simulink model "Spacecraft_ADCS (1)"  (R2017a)
settings: Solver=ode45  StartTime=0.0  StopTime=1000  RelTol=1e-7
values from neighbouring files (symbols this model uses):
  adr = ADRblockGen(w,m,3)    [Example__simulaltion (1).m]    (also in Example__simulaltion.m; WBC_setup (1).m)
  adr2 = ADRblockGen(w2,m,3)    [WBC_setup (1).m]
  aerodrag_A_d = 0.2*0.1*sqrt(2)    [Satellite_Setup_Sun_Pointing (1).m]    (also in Satellite_Setup_Sun_Pointing.m; Satellite_setup_ZenithPointing (1).m; Satellite_setup_ZenithPointing.m)
  aerodrag_c_p = 0.02*[1;1;1]    [Satellite_Setup_Sun_Pointing (1).m]    (also in Satellite_Setup_Sun_Pointing.m; Satellite_setup_ZenithPointing (1).m; Satellite_setup_ZenithPointing.m)
  distrej = 0    [Example__simulaltion (1).m]    (also in Example__simulaltion.m; WBC_setup (1).m = 1)
  I = diag([Ixx;Iyy;Izz])    [Satellite_Setup_Sun_Pointing (1).m]    (also in Satellite_Setup_Sun_Pointing.m; Satellite_setup_ZenithPointing (1).m; Satellite_setup_ZenithPointing.m)
  igrf_L = 10    [Satellite_Setup_Sun_Pointing (1).m]    (also in Satellite_Setup_Sun_Pointing.m; Satellite_setup_ZenithPointing (1).m; Satellite_setup_ZenithPointing.m)
  igrf_tol = 1e-9    (= 1e-09)    [Satellite_Setup_Sun_Pointing (1).m]    (also in Satellite_Setup_Sun_Pointing.m; Satellite_setup_ZenithPointing (1).m; Satellite_setup_ZenithPointing.m)
  k = 1e-9    (= 1e-09)    [Example__simulaltion (1).m]    (also in Example__simulaltion.m; WBC_setup (1).m = 5e-09)
  k2 = 5e-9    (= 5e-09)    [WBC_setup (1).m]
  kd = 6e-4    (= 0.0006)    [Example__simulaltion (1).m]    (also in Example__simulaltion.m; PD_SunPoint_setup (1).m = 2; PD_zenith_setup (1).m = 0.0002; PD_zenith_setup.m = 0.0002)
  kp = 5e-9    (= 5e-09)    [Example__simulaltion (1).m]    (also in Example__simulaltion.m; PD_SunPoint_setup (1).m = 0.0006; PD_zenith_setup (1).m = 1.6e-07; PD_zenith_setup.m = 1.6e-07)
  mass = 2.6    [Satellite_Setup_Sun_Pointing (1).m]    (also in Satellite_Setup_Sun_Pointing.m; Satellite_setup_ZenithPointing (1).m; Satellite_setup_ZenithPointing.m)
  nA = [nAx,nAy,nAz]    [Actuator_def.m]
  omega_orbit = [0;-7.67/(401.1+6371);0]    [Satellite_Setup_Sun_Pointing (1).m]    (also in Satellite_Setup_Sun_Pointing.m; Satellite_setup_ZenithPointing (1).m; Satellite_setup_ZenithPointing.m)
  q_ref = q_3_ref    [Example__simulaltion (1).m]    (also in Example__simulaltion.m)
  x_0 = transpose([wb_bi_init,qb_i_init])    [Example__simulaltion (1).m]    (also in Example__simulaltion.m; Satellite_Setup_Sun_Pointing (1).m = [transpose(wb_bi_init),qb_i_init]; Satellite_Setup_Sun_Pointing.m = [transpose(wb_bi_init),qb_i_init]; Satellite_setup_ZenithPointing (1).m = [(wb_bi_init),qb_i_init])
  x_orbit_init = [long_init,lat_init,altitude,qb_o_init,qo_i_init]    [Example__simulaltion (1).m]    (also in Example__simulaltion.m; Satellite_Setup_Sun_Pointing (1).m; Satellite_Setup_Sun_Pointing.m; Satellite_setup_ZenithPointing (1).m)
undefined symbols (not defined in the file or in its folder): i_coil, igrf_G, igrf_H, k_bd, m_coil, SkewSym, T_act
libraries: cstblocks x24, vrlib x8, sharedtransform x1
settings Model: Creator=joseph_thompson  LastModifiedBy=joseph_thompson

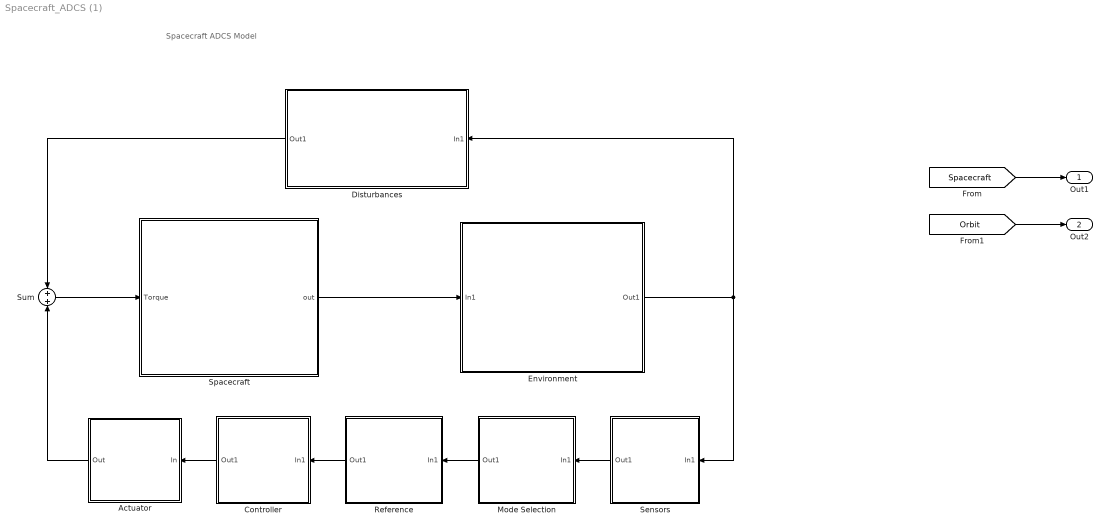
== system Spacecraft_ADCS (1) ==
  note: Spacecraft ADCS Model
  Actuator : Subsystem
  Controller : Subsystem
  Disturbances : Subsystem
  Environment : Subsystem
  Mode Selection : Subsystem
  Reference : Subsystem
  Sensors : Subsystem
  Spacecraft : Subsystem  VariantControl=Variant1
  Sum : Sum
  Out1 : Outport
  Out2 : Outport  Port=2
  wires:
  Spacecraft/1(out) -> Environment/1(In1)
  Environment/1(Out1) -> Disturbances/1(In1), Sensors/1(In1)
  Sensors/1(Out1) -> Mode Selection/1(In1)
  Mode Selection/1(Out1) -> Reference/1(In1)
  Actuator/1(Out) -> Sum/2
  Reference/1(Out1) -> Controller/1(In1)
  Controller/1(Out1) -> Actuator/1(In)
  [Spacecraft] -> Out1/1
  [Orbit] -> Out2/1
  Disturbances/1(Out1) -> Sum/1
  Sum/1 -> Spacecraft/1(Torque)

== system Spacecraft_ADCS (1)/Actuator ==
  In : Inport
  Variant Subsystem : Subsystem  Variant=on
  Out : Outport
  wires:
  In/1 -> Variant Subsystem/1(In1)
  Variant Subsystem/1(Out1) -> Out/1

== system Spacecraft_ADCS (1)/Controller ==
  In1 : Inport
  Add : Sum
  Bus Creator : BusCreator  Inputs=2
  Bus Selector : BusSelector  OutputSignals=q_ref,sensor_values,adcs_mode
  Controller : Subsystem  Commented=on  Variant=on
  No Control : Subsystem  TreatAsAtomicUnit=on
  PD : Subsystem  TreatAsAtomicUnit=on
  Switch Case : SwitchCase  CaseConditions={0,1,2,3}  ShowDefaultCase=off
  Out1 : Outport
  wires:
  In1/1 -> Bus Selector/1
  Bus Selector/1 -> Bus Creator/1  "<q_ref>"
  Bus Selector/2 -> Bus Creator/2  "<sensor_values>"
  Bus Creator/1 -> PD/1(In1), No Control/1(In1)
  Bus Selector/3 -> Switch Case/1  "<adcs_mode>"
  Switch Case/2 -> PD/Action
  Switch Case/4 -> No Control/Action
  No Control/1(Out1) -> Add/2
  Add/1 -> Out1/1
  PD/1(Out1) -> Add/1

== system Spacecraft_ADCS (1)/Disturbances ==
  In1 : Inport
  Bus Selector : BusSelector  OutputSignals=orbital_dynamics.qb_o,spacecraft_dynamics.omega_b_inert
  Constant : Constant  Value=7.2157
  Constant1 : Constant  Value=omega_orbit
  Constant2 : Constant  Value=[0,0,0]
  Constant3 : Constant  Value=[0,0,0]
  Level-2 MATLAB S-Function : M-S-Function  FunctionName=gravityGradientSfun
      mask Display:
      | disp('Gravity\n gradient')
      | port_label('input',1,'qb_o')
      | port_label('input',2,'omega orbit')
      | port_label('output',1,'T_b')
  Level-2 MATLAB S-Function1 : M-S-Function  FunctionName=aeroDragSfun  Parameters=I,mass,aerodrag_c_p,aerodrag_A_d  mask{Parameter1=I, Parameter2=mass, Parameter3=aerodrag_c_p, Parameter4=aerodrag_A_d}
      mask prompts: Parameter1 "Inertia"; Parameter2 "Mass"; Parameter3 "COP vector"; Parameter4 "Area"
      mask Display:
      | disp('Aerodynamic\n drag')
      | port_label('input',1,'qb_o')
      | port_label('input',2,'omega orbit')
      | port_label('input',3,'Local atmosph. vel')
      | port_label('output',1,'T_b')
  Total Dist. Torque : Sum  Inputs=++++
  Out1 : Outport
  wires:
  Constant2/1 -> Total Dist. Torque/4  "internal_magnetic_dipole_torque"
  Constant3/1 -> Total Dist. Torque/3  "solar_radiation_pressure_torque"
  Bus Selector/2 -> Level-2 MATLAB S-Function1/4  "<omega_b_inert>"
  Constant/1 -> Level-2 MATLAB S-Function1/3
  Constant1/1 -> Level-2 MATLAB S-Function/2, Level-2 MATLAB S-Function1/2  "<omega_orbit>"
  Bus Selector/1 -> Level-2 MATLAB S-Function/1, Level-2 MATLAB S-Function1/1  "<qb_o>"
  In1/1 -> Bus Selector/1
  Level-2 MATLAB S-Function1/1 -> Total Dist. Torque/2  "aero_drag_torque"
  Level-2 MATLAB S-Function/1 -> Total Dist. Torque/1  "gravity_gradient_torque"
  Total Dist. Torque/1 -> Out1/1  "total_dist_torque"

== system Spacecraft_ADCS (1)/Environment ==
  In1 : Inport
  Bus Creator : BusCreator  Inputs=3
  Bus Creator1 : BusCreator  Inputs=1
  Bus Selector : BusSelector  OutputSignals=orbital_dynamics.LongLatAlt,spacecraft_dynamics,orbital_dynamics
  Constant : Constant  Value=0
  Level-2 MATLAB S-Function : M-S-Function  FunctionName=IGRFSfun  Parameters=igrf_L,igrf_tol,igrf_G,igrf_H  mask{Parameter1=igrf_L, Parameter2=igrf_tol, Parameter3=igrf_G, Parameter4=igrf_H}
      mask prompts: Parameter1 "L"; Parameter2 "tolerance"; Parameter3 "G_coefs"; Parameter4 "H_coefs"
      mask Display:
      | disp('IGRF 11\n  Geomagnetic reference')
      | port_label('input',1,'LLA')
      | port_label('output',1,'real B')
  Out1 : Outport
  wires:
  Level-2 MATLAB S-Function/1 -> Bus Creator1/1  "B_real"
  Constant/1 -> Level-2 MATLAB S-Function/2  "B_real"
  Bus Creator/1 -> Out1/1
  Bus Selector/1 -> Level-2 MATLAB S-Function/1  "<LongLatAlt>"
  In1/1 -> Bus Selector/1  "Dyn_out"
  Bus Selector/2 -> Bus Creator/1  "<spacecraft_dynamics>"
  Bus Selector/3 -> Bus Creator/2  "<orbital_dynamics>"
  Bus Creator1/1 -> Bus Creator/3  "Environment"

== system Spacecraft_ADCS (1)/Mode Selection ==
  In1 : Inport
  Bus Creator : BusCreator  Inputs=2
  Constant : Constant
  Out1 : Outport
  wires:
  Bus Creator/1 -> Out1/1
  In1/1 -> Bus Creator/1  "sensor_values"
  Constant/1 -> Bus Creator/2  "adcs_mode"

== system Spacecraft_ADCS (1)/Reference ==
  In1 : Inport
  Bus Creator : BusCreator  Inputs=3
  Bus Selector : BusSelector  OutputSignals=sensor_values,adcs_mode
  Constant : Constant  Value=q_ref
  Out1 : Outport
  wires:
  Constant/1 -> Bus Creator/3  "q_ref"
  In1/1 -> Bus Selector/1
  Bus Selector/1 -> Bus Creator/1  "<sensor_values>"
  Bus Selector/2 -> Bus Creator/2  "<adcs_mode>"
  Bus Creator/1 -> Out1/1

== system Spacecraft_ADCS (1)/Sensors ==
  In1 : Inport
  Bus Creator : BusCreator  Inputs=6
  Bus Selector : BusSelector  OutputSignals=spacecraft_dynamics.omega_b_inert,spacecraft_dynamics.qb_i,orbital_dynamics.LongLatAlt,orbital_dynamics.qb_o,orbital_dynamics.qo_i,Environment.B_real
  Out1 : Outport
  wires:
  In1/1 -> Bus Selector/1  "Actual_Values"
  Bus Selector/1 -> Bus Creator/1  "<omega_b_inert>"
  Bus Selector/2 -> Bus Creator/2  "<qb_i>"
  Bus Selector/4 -> Bus Creator/4  "<qb_o>"
  Bus Selector/5 -> Bus Creator/5  "<qo_i>"
  Bus Selector/6 -> Bus Creator/6  "<B_real>"
  Bus Selector/3 -> Bus Creator/3  "<LongLatAlt>"
  Bus Creator/1 -> Out1/1

== system Spacecraft_ADCS (1)/Spacecraft ==
  Torque : Inport
  Bus Creator1 : BusCreator  Inputs=3
  Bus Creator2 : BusCreator  Inputs=2
  Bus Selector2 : BusSelector  OutputSignals=omega_b_inert
  Orbit Propagation : M-S-Function  FunctionName=OrbitSfun  Parameters=x_orbit_init,omega_orbit  mask{Parameter1=x_orbit_init, Parameter2=omega_orbit}
      mask prompts: Parameter1 "Initial orbit param"; Parameter2 "orbit angular velocity"
      mask DialogControl Control8 Prompt: Orbit properties
      mask Display:
      | disp('Orbital Parameters')
      | port_label('input',1,'ang vel')
      | port_label('output',1,'LLA')
      | port_label('output',2,'qb_o')
      | port_label('output',3,'qo_i')
  Spacecraft Rotational Dynamics : Subsystem  Variant=on  VariantControl=Variant1  OverrideUsingVariant=Variant1
  out : Outport
  tag scope: Orbit=global, Spacecraft=global
  wires:
  Orbit Propagation/3 -> Bus Creator1/3  "qo_i"
  Orbit Propagation/2 -> Bus Creator1/2  "qb_o"
  Orbit Propagation/1 -> Bus Creator1/1  "LongLatAlt"
  Bus Creator1/1 -> [Orbit], Bus Creator2/2  "orbital_dynamics"
  Bus Creator2/1 -> out/1
  Torque/1 -> Spacecraft Rotational Dynamics/1("In1 ")  "T_total"
  Spacecraft Rotational Dynamics/1(" Out1") -> [Spacecraft], Bus Selector2/1, Bus Creator2/1
  Bus Selector2/1 -> Orbit Propagation/1  "<omega_b_inert>"

== system Spacecraft_ADCS (1)/Actuator/Variant Subsystem ==
  note: 1) Only subsystems can be added as variant choices at this level
      | 2) Blocks cannot be connected at this level as connectivity is
      | automatically determined at simulation, based on the active variant
  In1 : Inport
  2 coil dipole : Subsystem  VariantControl=ActType==5
  3 coil dipole : Subsystem  VariantControl=ActType==4
  Ideal : Subsystem  VariantControl=ActType==1
  Three Axis MagTorq : Subsystem  VariantControl=ActType==2
  Two Axis MagTorq : Subsystem  VariantControl=ActType==3
  Out1 : Outport

== system Spacecraft_ADCS (1)/Controller/Controller ==
  note: 1) Only subsystems can be added as variant choices at this level
      | 2) Blocks cannot be connected at this level as connectivity is
      | automatically determined at simulation, based on the active variant
  bus in : Inport
  B dot : Subsystem  VariantControl=CtrlType==4
  PD : Subsystem  VariantControl=CtrlType==2
  PD Zenith : Subsystem  VariantControl=CtrlType==3
  WBC : Subsystem  VariantControl=CtrlType==1
  WBC detumble : Subsystem  VariantControl=CtrlType==5
  no control : Subsystem  VariantControl=CtrlType==0
  bus out : Outport

== system Spacecraft_ADCS (1)/Controller/No Control ==
  In1 : Inport
  Action Port : ActionPort  ActionType=case
  Constant : Constant  Value=[0,0,0]
  Out1 : Outport
  wires:
  Constant/1 -> Out1/1

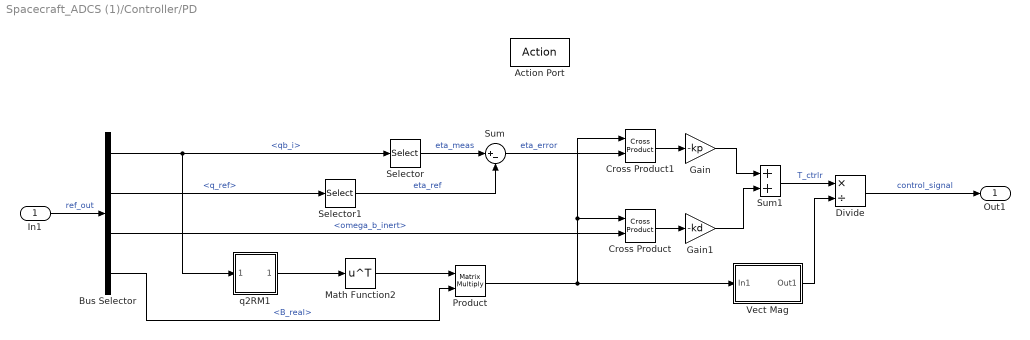
== system Spacecraft_ADCS (1)/Controller/PD ==
  In1 : Inport
  Action Port : ActionPort  ActionType=case
  Bus Selector : BusSelector  OutputSignals=sensor_values.qb_i,q_ref,sensor_values.omega_b_inert,sensor_values.B_real
  Cross Product : vrlib/Utilities/Cross Product
      settings: SourceProductBaseCode=VR
  Cross Product1 : vrlib/Utilities/Cross Product
      settings: SourceProductBaseCode=VR
  Divide : Product  Inputs=*/
  Gain : Gain  Gain=-kp
  Gain1 : Gain  Gain=-kd
  Math Function2 : Math  Operator=transpose  SaturateOnIntegerOverflow=on
  Product : Product  Multiplication=Matrix(*)
  Selector : Selector  InputPortWidth=4  IndexOptions=Index vector (dialog)  Indices=[2 3 4]  OutputSizes=1
  Selector1 : Selector  InputPortWidth=4  IndexOptions=Index vector (dialog)  Indices=[2 3 4]  OutputSizes=1
  Sum : Sum  Inputs=|+-
  Sum1 : Sum
  Vect Mag : Subsystem
  q2RM1 : Subsystem
  Out1 : Outport
  wires:
  Cross Product/1 -> Gain1/1
  Bus Selector/2 -> Selector1/1  "<q_ref>"
  Bus Selector/4 -> Product/2  "<B_real>"
  Divide/1 -> Out1/1  "control_signal"
  In1/1 -> Bus Selector/1  "ref_out"
  q2RM1/1(Out1) -> Math Function2/1
  Gain1/1 -> Sum1/2
  Product/1 -> Vect Mag/1(In1), Cross Product/1, Cross Product1/1
  Gain/1 -> Sum1/1
  Sum/1 -> Cross Product1/2  "eta_error"
  Bus Selector/1 -> Selector/1, q2RM1/1(In1)  "<qb_i>"
  Bus Selector/3 -> Cross Product/2  "<omega_b_inert>"
  Sum1/1 -> Divide/1  "T_ctrlr"
  Selector1/1 -> Sum/2  "eta_ref"
  Math Function2/1 -> Product/1
  Vect Mag/1(Out1) -> Divide/2
  Cross Product1/1 -> Gain/1
  Selector/1 -> Sum/1  "eta_meas"

== system Spacecraft_ADCS (1)/Spacecraft/Spacecraft Rotational Dynamics ==
  "In1 " : Inport
  Subsystem : Subsystem  VariantControl=Variant1
  " Out1" : Outport

== system Spacecraft_ADCS (1)/Actuator/Variant Subsystem/2 coil dipole ==
  In1 : Inport
  B vect from inert frm to body frm : Subsystem
  Bus Assignment : BusAssignment  AssignedSignals=m_coil,T_act,i_coil
  Bus Selector : BusSelector  OutputSignals=m_b,Sensor_Values.B_i,Sensor_Values.qb_i
  Constant : Constant  Value=nA
  Constant3 : Constant  Value=0
  Cross Product : vrlib/Utilities/Cross Product
      settings: SourceProductBaseCode=VR
  Divide : Product  Inputs=*/
  Mux1 : Mux  Inputs=2
  Saturation : Saturate  UpperLimit=0.24  LowerLimit=-0.24
  Selector : Selector  InputPortWidth=3  IndexOptions=Index vector (dialog)  Indices=[1 2]  OutputSizes=1
  Out1 : Outport
  wires:
  B vect from inert frm to body frm/1(B_b) -> Cross Product/2
  Bus Selector/3 -> B vect from inert frm to body frm/2(q)  "<qb_i>"
  Bus Selector/2 -> B vect from inert frm to body frm/1(B_i)  "<B_i>"
  Constant3/1 -> Mux1/2
  Selector/1 -> Mux1/1
  Mux1/1 -> Saturation/1
  In1/1 -> Bus Assignment/1, Bus Selector/1  "Ctrlr_out"
  Bus Assignment/1 -> Out1/1
  Cross Product/1 -> Bus Assignment/3  "T_act"
  Bus Selector/1 -> Selector/1  "<m_b>"
  Divide/1 -> Bus Assignment/4  "i_coil"
  Constant/1 -> Divide/2
  Saturation/1 -> Cross Product/1, Divide/1, Bus Assignment/2

== system Spacecraft_ADCS (1)/Actuator/Variant Subsystem/3 coil dipole ==
  In1 : Inport
  B vect from inert frm to body frm : Subsystem
  Bus Assignment : BusAssignment  AssignedSignals=m_coil,T_act,i_coil
  Bus Selector : BusSelector  OutputSignals=m_b,Sensor_Values.B_i,Sensor_Values.qb_i
  Constant : Constant  Value=nA
  Cross Product : vrlib/Utilities/Cross Product
      settings: SourceProductBaseCode=VR
  Divide : Product  Inputs=*/
  Saturation : Saturate  UpperLimit=0.24  LowerLimit=-0.24
  Out1 : Outport
  wires:
  Bus Assignment/1 -> Out1/1
  B vect from inert frm to body frm/1(B_b) -> Cross Product/2
  Bus Selector/3 -> B vect from inert frm to body frm/2(q)  "<qb_i>"
  Bus Selector/2 -> B vect from inert frm to body frm/1(B_i)  "<B_i>"
  In1/1 -> Bus Assignment/1, Bus Selector/1  "Ctrlr_out"
  Cross Product/1 -> Bus Assignment/3  "T_act"
  Bus Selector/1 -> Saturation/1  "<m_b>"
  Divide/1 -> Bus Assignment/4  "i_coil"
  Constant/1 -> Divide/2
  Saturation/1 -> Cross Product/1, Divide/1, Bus Assignment/2

== system Spacecraft_ADCS (1)/Actuator/Variant Subsystem/Ideal ==
  In1 : Inport
  Out1 : Outport
  wires:
  In1/1 -> Out1/1  "Ctrlr_out"

== system Spacecraft_ADCS (1)/Actuator/Variant Subsystem/Three Axis MagTorq ==
  In1 : Inport
  B vect from inert frm to body frm : Subsystem
  B vect from inert frm to body frm1 : Subsystem
  Bus Assignment : BusAssignment  AssignedSignals=T_act,m_coil,i_coil
  Bus Selector : BusSelector  OutputSignals=T_ctrlr,Actual_Values.B_i,Sensor_Values.B_i,Sensor_Values.qb_i
  Level-2 MATLAB S-Function : M-S-Function  FunctionName=Magtorq2Sfun  Parameters=nAx, nAy, nAz
  Out1 : Outport
  wires:
  B vect from inert frm to body frm1/1(B_b) -> ?
  B vect from inert frm to body frm/1(B_b) -> ?
  Bus Selector/4 -> B vect from inert frm to body frm/1(q), B vect from inert frm to body frm1/1(q)  "<qb_i>"
  Level-2 MATLAB S-Function/3 -> Bus Assignment/4  "i_coil"
  Level-2 MATLAB S-Function/2 -> Bus Assignment/3  "m_coil"
  Bus Selector/2 -> B vect from inert frm to body frm/2(B_i), Level-2 MATLAB S-Function/2  "<B_i>"
  Bus Selector/1 -> Level-2 MATLAB S-Function/1  "<T_ctrlr>"
  Level-2 MATLAB S-Function/1 -> Bus Assignment/2  "T_act"
  Bus Selector/3 -> B vect from inert frm to body frm1/2(B_i), Level-2 MATLAB S-Function/3  "<B_i>"
  Bus Assignment/1 -> Out1/1
  In1/1 -> Bus Selector/1, Bus Assignment/1

== system Spacecraft_ADCS (1)/Actuator/Variant Subsystem/Two Axis MagTorq ==
  In1 : Inport
  Bus Creator : BusCreator  Inputs=4
  Bus Selector : BusSelector  OutputSignals=T_ctrlr,ref_out.Mode_select_out.Sensor_out.Enviro_out.B_real,ref_out.Mode_select_out.Sensor_out.Sensor_values.B_real
  Level-2 MATLAB S-Function : M-S-Function  FunctionName=MagtorqSfun
  Selector : Selector  InputPortWidth=3  IndexOptions=Index vector (dialog)  Indices=[1 2]  OutputSizes=1
  Out1 : Outport
  wires:
  ? -> Bus Creator/4  "i_coil"
  Level-2 MATLAB S-Function/2 -> Bus Creator/3
  Selector/1 -> Bus Creator/2  "m_coils"
  Level-2 MATLAB S-Function/1 -> Selector/1
  Bus Selector/2 -> Level-2 MATLAB S-Function/2  "<B_real>"
  Bus Selector/1 -> Level-2 MATLAB S-Function/1  "<T_ctrlr>"
  Bus Selector/3 -> Level-2 MATLAB S-Function/3  "<B_real>"
  Bus Creator/1 -> Out1/1
  In1/1 -> Bus Creator/1, Bus Selector/1

== system Spacecraft_ADCS (1)/Controller/Controller/B dot ==
  bus in : Inport
  Bus Creator : BusCreator  Inputs=2
  Bus Selector : BusSelector  OutputSignals=signal1.Sensor_out.Sensor_Values.qb_i,q_ref,signal1.Sensor_out.Sensor_Values.omega_b_inert,signal1.Sensor_out.Sensor_Values.B_real,signal1.Sensor_out.Actual_Values.Dyn_out.qb_o
  Derivative : Derivative
  Gain : Gain  Gain=-k_bd
  bus out : Outport
  wires:
  Gain/1 -> Bus Creator/2  "T_ctrlr"
  Derivative/1 -> Gain/1
  Bus Selector/4 -> Derivative/1  "<B_real>"
  bus in/1 -> Bus Selector/1, Bus Creator/1  "ref_out"
  Bus Creator/1 -> bus out/1

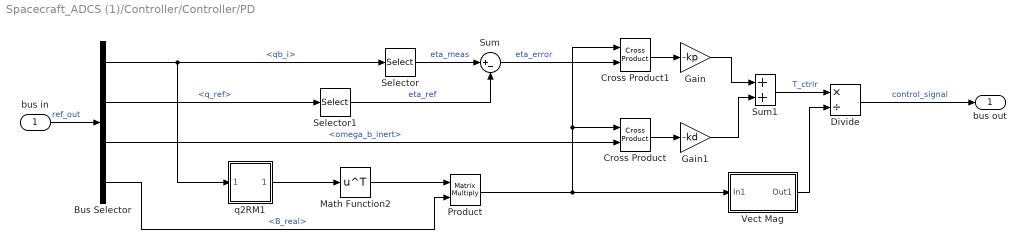
== system Spacecraft_ADCS (1)/Controller/Controller/PD ==
  bus in : Inport
  Bus Selector : BusSelector  OutputSignals=sensor_values.qb_i,q_ref,sensor_values.omega_b_inert,sensor_values.B_real
  Cross Product : vrlib/Utilities/Cross Product
      settings: SourceProductBaseCode=VR
  Cross Product1 : vrlib/Utilities/Cross Product
      settings: SourceProductBaseCode=VR
  Divide : Product  Inputs=*/
  Gain : Gain  Gain=-kp
  Gain1 : Gain  Gain=-kd
  Math Function2 : Math  Operator=transpose  SaturateOnIntegerOverflow=on
  Product : Product  Multiplication=Matrix(*)
  Selector : Selector  InputPortWidth=4  IndexOptions=Index vector (dialog)  Indices=[2 3 4]  OutputSizes=1
  Selector1 : Selector  InputPortWidth=4  IndexOptions=Index vector (dialog)  Indices=[2 3 4]  OutputSizes=1
  Sum : Sum  Inputs=|+-
  Sum1 : Sum
  Vect Mag : Subsystem
  q2RM1 : Subsystem
  bus out : Outport
  wires:
  Bus Selector/3 -> Cross Product/2  "<omega_b_inert>"
  Sum1/1 -> Divide/1  "T_ctrlr"
  q2RM1/1(Out1) -> Math Function2/1
  Math Function2/1 -> Product/1
  Bus Selector/4 -> Product/2  "<B_real>"
  Cross Product/1 -> Gain1/1
  Cross Product1/1 -> Gain/1
  Bus Selector/1 -> Selector/1, q2RM1/1(In1)  "<qb_i>"
  Sum/1 -> Cross Product1/2  "eta_error"
  Vect Mag/1(Out1) -> Divide/2
  Product/1 -> Vect Mag/1(In1), Cross Product/1, Cross Product1/1
  Gain1/1 -> Sum1/2
  Gain/1 -> Sum1/1
  Selector1/1 -> Sum/2  "eta_ref"
  Selector/1 -> Sum/1  "eta_meas"
  Bus Selector/2 -> Selector1/1  "<q_ref>"
  bus in/1 -> Bus Selector/1  "ref_out"
  Divide/1 -> bus out/1  "control_signal"

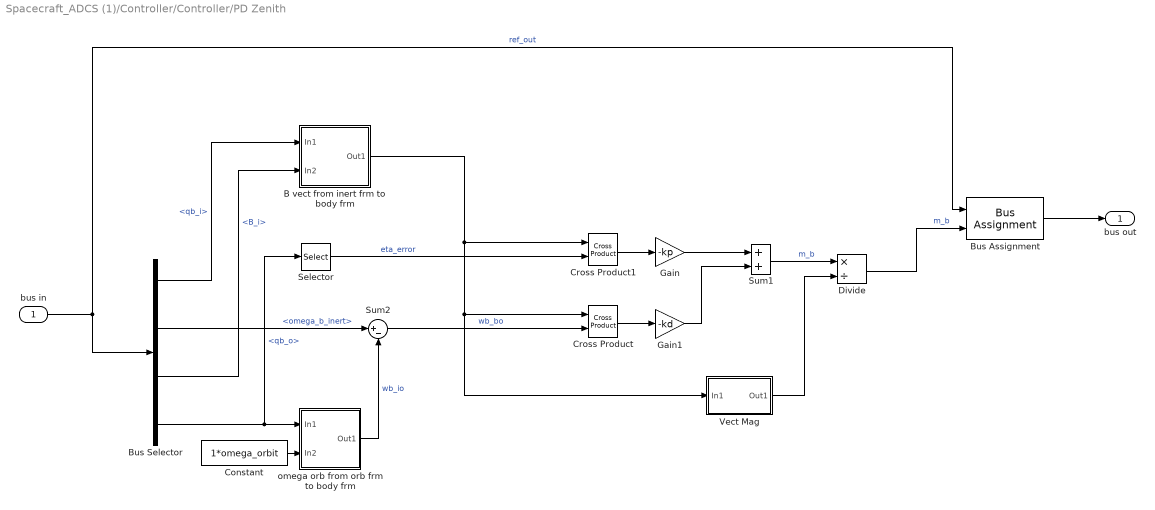
== system Spacecraft_ADCS (1)/Controller/Controller/PD Zenith ==
  bus in : Inport
  B vect from inert frm to body frm : Subsystem
  Bus Assignment : BusAssignment  AssignedSignals=m_b
  Bus Selector : BusSelector  OutputSignals=Sensor_Values.qb_i,Sensor_Values.omega_b_inert,Sensor_Values.B_i,Actual_Values.qb_o
  Constant : Constant  Value=1*omega_orbit
  Cross Product : vrlib/Utilities/Cross Product
      settings: SourceProductBaseCode=VR
  Cross Product1 : vrlib/Utilities/Cross Product
      settings: SourceProductBaseCode=VR
  Divide : Product  Inputs=*/
  Gain : Gain  Gain=-kp
  Gain1 : Gain  Gain=-kd
  Selector : Selector  InputPortWidth=4  IndexOptions=Index vector (dialog)  Indices=[2 3 4]  OutputSizes=1
  Sum1 : Sum
  Sum2 : Sum  Inputs=|+-
  Vect Mag : Subsystem
  omega orb from orb frm to body frm : Subsystem
  bus out : Outport
  wires:
  Bus Selector/3 -> B vect from inert frm to body frm/2(In2)  "<B_i>"
  Bus Selector/1 -> B vect from inert frm to body frm/1(In1)  "<qb_i>"
  B vect from inert frm to body frm/1(Out1) -> Cross Product1/1, Cross Product/1, Vect Mag/1(In1)
  omega orb from orb frm to body frm/1(Out1) -> Sum2/2  "wb_io"
  Constant/1 -> omega orb from orb frm to body frm/2(In2)
  Bus Selector/4 -> omega orb from orb frm to body frm/1(In1), Selector/1  "<qb_o>"
  Bus Selector/2 -> Sum2/1  "<omega_b_inert>"
  bus in/1 -> Bus Selector/1, Bus Assignment/1  "ref_out"
  Gain/1 -> Sum1/1
  Gain1/1 -> Sum1/2
  Bus Assignment/1 -> bus out/1
  Vect Mag/1(Out1) -> Divide/2
  Sum2/1 -> Cross Product/2  "wb_bo"
  Sum1/1 -> Divide/1  "m_b"
  Selector/1 -> Cross Product1/2  "eta_error"
  Cross Product/1 -> Gain1/1
  Cross Product1/1 -> Gain/1
  Divide/1 -> Bus Assignment/2  "m_b"

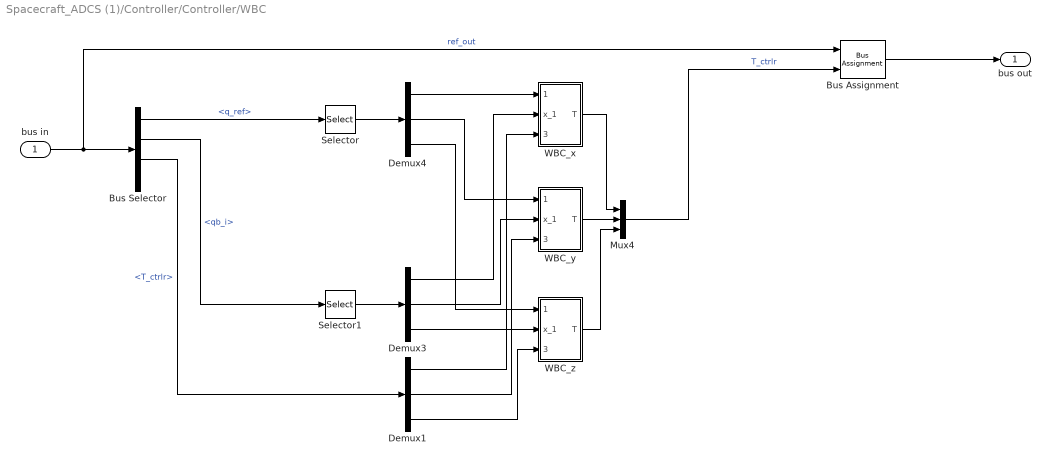
== system Spacecraft_ADCS (1)/Controller/Controller/WBC ==
  bus in : Inport
  Bus Assignment : BusAssignment  AssignedSignals=T_ctrlr
  Bus Selector : BusSelector  OutputSignals=q_ref,Sensor_Values.qb_i,T_ctrlr,Sensor_Values.B_i
  Demux1 : Demux  Outputs=3
  Demux3 : Demux  Outputs=3
  Demux4 : Demux  Outputs=3
  Mux4 : Mux  Inputs=3
  Selector : Selector  InputPortWidth=4  IndexOptions=Index vector (dialog)  Indices=[2 3 4]  OutputSizes=1
  Selector1 : Selector  InputPortWidth=4  IndexOptions=Index vector (dialog)  Indices=[2 3 4]  OutputSizes=1
  WBC_x : Subsystem
  WBC_y : Subsystem
  WBC_z : Subsystem
  bus out : Outport
  wires:
  Selector/1 -> Demux4/1
  Bus Assignment/1 -> bus out/1
  Bus Selector/2 -> Selector1/1  "<qb_i>"
  Bus Selector/1 -> Selector/1  "<q_ref>"
  bus in/1 -> Bus Selector/1, Bus Assignment/1  "ref_out"
  Selector1/1 -> Demux3/1
  Demux4/2 -> WBC_y/1(x_0_ref)
  Demux4/3 -> WBC_z/1(x_0_ref)
  Demux4/1 -> WBC_x/1(x_0_ref)
  Demux1/3 -> WBC_z/3(T_meas)
  Demux1/2 -> WBC_y/3(T_meas)
  Demux1/1 -> WBC_x/3(T_meas)
  Bus Selector/3 -> Demux1/1  "<T_ctrlr>"
  Demux3/1 -> WBC_x/2(x_1)
  Demux3/2 -> WBC_y/2(x_1)
  WBC_x/1(T) -> Mux4/1
  WBC_z/1(T) -> Mux4/3
  Mux4/1 -> Bus Assignment/2  "T_ctrlr"
  WBC_y/1(T) -> Mux4/2
  Demux3/3 -> WBC_z/2(x_1)

== system Spacecraft_ADCS (1)/Controller/Controller/WBC detumble ==
  bus in : Inport
  Bus Creator : BusCreator  Inputs=2
  Bus Selector : BusSelector  OutputSignals=q_ref,signal1.Sensor_out.Sensor_values.omega_b_inert,signal1.Sensor_out.Enviro_out.Dyn_out.T_ctrlr
  Demux1 : Demux  Outputs=3
  Demux3 : Demux  Outputs=3
  Demux4 : Demux  Outputs=3
  Mux4 : Mux  Inputs=3
  Quaternions to Rotation Angles : sharedtransform/Quaternions to Rotation Angles  Commented=on  rotationOrder=ZYX
      settings: SourceProductBaseCode=AE
  Vector Mag1 : Subsystem  Commented=on
  WBC_x : Subsystem
  WBC_y : Subsystem
  WBC_z : Subsystem
  bus out : Outport
  wires:
  Demux3/3 -> WBC_z/2(x_1)
  WBC_y/1(T) -> Mux4/2
  Mux4/1 -> Bus Creator/2  "T_ctrlr"
  WBC_z/1(T) -> Mux4/3
  WBC_x/1(T) -> Mux4/1
  Demux3/2 -> WBC_y/2(x_1)
  Demux3/1 -> WBC_x/2(x_1)
  Bus Selector/3 -> Demux1/1  "<T_ctrlr>"
  Demux1/1 -> WBC_x/3(T_meas)
  Demux1/2 -> WBC_y/3(T_meas)
  Demux1/3 -> WBC_z/3(T_meas)
  Demux4/1 -> WBC_x/1(x_0_ref)
  Demux4/3 -> WBC_z/1(x_0_ref)
  Demux4/2 -> WBC_y/1(x_0_ref)
  bus in/1 -> Bus Creator/1, Bus Selector/1  "ref_out"
  Bus Selector/1 -> ?  "<q_ref>"
  Bus Selector/2 -> Demux3/1  "<omega_b_inert>"
  Bus Creator/1 -> bus out/1
  ? -> Demux4/1

== system Spacecraft_ADCS (1)/Controller/Controller/no control ==
  bus in : Inport
  Bus : Subsystem  Commented=on
  Bus Creator : BusCreator  Inputs=2
  Constant : Constant  Value=[0;0;0]
  bus out : Outport
  wires:
  Bus Creator/1 -> bus out/1
  Constant/1 -> Bus Creator/2  "T_ctrlr"
  bus in/1 -> Bus Creator/1  "ref_out"

== system Spacecraft_ADCS (1)/Controller/PD/Vect Mag ==
  In1 : Inport
  Math Function : Math  Operator=square  SaturateOnIntegerOverflow=on
  Sqrt : Sqrt  SaturateOnIntegerOverflow=on
  Sum2 : Sum  Inputs=+
  Out1 : Outport
  wires:
  Sum2/1 -> Sqrt/1
  Math Function/1 -> Sum2/1
  In1/1 -> Math Function/1
  Sqrt/1 -> Out1/1

== system Spacecraft_ADCS (1)/Controller/PD/q2RM1 ==
  In1 : Inport
  Add : Sum
  Constant : Constant  Value=eye(3)
  Fcn : Fcn  Commented=on  Expr=SkewSym([u(1),u(2),u(3)])
  Gain : Gain  Gain=2
  Interpreted MATLAB Function : MATLABFcn  MATLABFcn=SkewSym([u(1),u(2),u(3)],1)  OutputDimensions=9
  Math Function : Math  Operator=square  SaturateOnIntegerOverflow=on
  Product : Product
  Reshape : Reshape  OutputDimensionality=Customize  OutputDimensions=[3,3]
  Selector : Selector  InputPortWidth=4  IndexOptions=Index vector (dialog)  Indices=[1]  OutputSizes=1
  Selector1 : Selector  InputPortWidth=4  IndexOptions=Index vector (dialog)  Indices=[2 3 4]  OutputSizes=1
  Sum : Sum
  Out1 : Outport
  wires:
  Interpreted MATLAB Function/1 -> Reshape/1
  Add/1 -> Out1/1
  Constant/1 -> Add/1
  Gain/1 -> Add/2
  Sum/1 -> Gain/1
  Math Function/1 -> Sum/2
  Product/1 -> Sum/1
  Selector1/1 -> Interpreted MATLAB Function/1
  Selector/1 -> Product/1
  Reshape/1 -> Product/2, Math Function/1
  In1/1 -> Selector1/1, Selector/1

== system Spacecraft_ADCS (1)/Spacecraft/Spacecraft Rotational Dynamics/Subsystem ==
  In1 : Inport
  Bus Creator : BusCreator  Inputs=2
  Spacecraft Rotational Dynamics : M-S-Function  FunctionName=CubeSatSfun  Parameters=x_0,I  mask{Parameter2=x_0, Parameter3=I}
      mask prompts: Parameter2 "x_0"; Parameter3 "I"
      mask DialogControl DescTextVar Prompt: Model of a rigid CubeSat. Model takes Torque about each axis as an input. The first output is the angular velocity of the sat wrt an inertial frame. The second output is the quaternion which represents the rotation between inertial and body fixed frames
      mask Display:
      | disp('Cube Sat Model')
      | port_label('input',1,'Torq')
      | port_label('output',1,'Ang Vel')
      | port_label('output',2,'Quat')
  Out1 : Outport
  wires:
  Spacecraft Rotational Dynamics/2 -> Bus Creator/2  "qb_i"
  Spacecraft Rotational Dynamics/1 -> Bus Creator/1  "omega_b_inert"
  In1/1 -> Spacecraft Rotational Dynamics/1
  Bus Creator/1 -> Out1/1  "spacecraft_dynamics"

== system Spacecraft_ADCS (1)/Actuator/Variant Subsystem/2 coil dipole/B vect from inert frm to body frm ==
  B_i : Inport
  q : Inport  Port=2
  Math Function2 : Math  Operator=transpose  SaturateOnIntegerOverflow=on
  Product : Product  Multiplication=Matrix(*)
  q2RM : Subsystem
  B_b : Outport
  wires:
  q2RM/1(Out1) -> Math Function2/1
  q/1 -> q2RM/1(In1)
  Math Function2/1 -> Product/1
  Product/1 -> B_b/1
  B_i/1 -> Product/2

== system Spacecraft_ADCS (1)/Actuator/Variant Subsystem/3 coil dipole/B vect from inert frm to body frm ==
  B_i : Inport
  q : Inport  Port=2
  Math Function2 : Math  Operator=transpose  SaturateOnIntegerOverflow=on
  Product : Product  Multiplication=Matrix(*)
  q2RM : Subsystem
  B_b : Outport
  wires:
  q2RM/1(Out1) -> Math Function2/1
  q/1 -> q2RM/1(In1)
  Math Function2/1 -> Product/1
  Product/1 -> B_b/1
  B_i/1 -> Product/2

== system Spacecraft_ADCS (1)/Actuator/Variant Subsystem/Three Axis MagTorq/B vect from inert frm to body frm ==
  q : Inport
  B_i : Inport  Port=2
  Math Function1 : Math  Operator=transpose  SaturateOnIntegerOverflow=on
  Product : Product  Multiplication=Matrix(*)
  q2RM2 : Subsystem
  B_b : Outport
  wires:
  B_i/1 -> Product/2
  Product/1 -> B_b/1
  Math Function1/1 -> Product/1
  q/1 -> q2RM2/1(In1)
  q2RM2/1(Out1) -> Math Function1/1

== system Spacecraft_ADCS (1)/Actuator/Variant Subsystem/Three Axis MagTorq/B vect from inert frm to body frm1 ==
  q : Inport
  B_i : Inport  Port=2
  Math Function1 : Math  Operator=transpose  SaturateOnIntegerOverflow=on
  Product1 : Product  Multiplication=Matrix(*)
  q2RM2 : Subsystem
  B_b : Outport
  wires:
  Product1/1 -> B_b/1
  q2RM2/1(Out1) -> Math Function1/1
  q/1 -> q2RM2/1(In1)
  Math Function1/1 -> Product1/1
  B_i/1 -> Product1/2

== system Spacecraft_ADCS (1)/Controller/Controller/PD/Vect Mag ==
  In1 : Inport
  Math Function : Math  Operator=square  SaturateOnIntegerOverflow=on
  Sqrt : Sqrt  SaturateOnIntegerOverflow=on
  Sum2 : Sum  Inputs=+
  Out1 : Outport
  wires:
  Sum2/1 -> Sqrt/1
  Math Function/1 -> Sum2/1
  In1/1 -> Math Function/1
  Sqrt/1 -> Out1/1

== system Spacecraft_ADCS (1)/Controller/Controller/PD/q2RM1 ==
  In1 : Inport
  Add : Sum
  Constant : Constant  Value=eye(3)
  Fcn : Fcn  Commented=on  Expr=SkewSym([u(1),u(2),u(3)])
  Gain : Gain  Gain=2
  Interpreted MATLAB Function : MATLABFcn  MATLABFcn=SkewSym([u(1),u(2),u(3)],1)  OutputDimensions=9
  Math Function : Math  Operator=square  SaturateOnIntegerOverflow=on
  Product : Product
  Reshape : Reshape  OutputDimensionality=Customize  OutputDimensions=[3,3]
  Selector : Selector  InputPortWidth=4  IndexOptions=Index vector (dialog)  Indices=[1]  OutputSizes=1
  Selector1 : Selector  InputPortWidth=4  IndexOptions=Index vector (dialog)  Indices=[2 3 4]  OutputSizes=1
  Sum : Sum
  Out1 : Outport
  wires:
  Interpreted MATLAB Function/1 -> Reshape/1
  Add/1 -> Out1/1
  Constant/1 -> Add/1
  Gain/1 -> Add/2
  Sum/1 -> Gain/1
  Math Function/1 -> Sum/2
  Product/1 -> Sum/1
  Selector1/1 -> Interpreted MATLAB Function/1
  Selector/1 -> Product/1
  Reshape/1 -> Product/2, Math Function/1
  In1/1 -> Selector1/1, Selector/1

== system Spacecraft_ADCS (1)/Controller/Controller/PD Zenith/B vect from inert frm to body frm ==
  In1 : Inport
  In2 : Inport  Port=2
  Math Function1 : Math  Operator=transpose  SaturateOnIntegerOverflow=on
  Product1 : Product  Multiplication=Matrix(*)
  q2RM2 : Subsystem
  Out1 : Outport
  wires:
  In2/1 -> Product1/2
  Math Function1/1 -> Product1/1
  In1/1 -> q2RM2/1(In1)
  q2RM2/1(Out1) -> Math Function1/1
  Product1/1 -> Out1/1

== system Spacecraft_ADCS (1)/Controller/Controller/PD Zenith/Vect Mag ==
  In1 : Inport
  Math Function : Math  Operator=square  SaturateOnIntegerOverflow=on
  Sqrt : Sqrt  SaturateOnIntegerOverflow=on
  Sum2 : Sum  Inputs=+
  Out1 : Outport
  wires:
  Sqrt/1 -> Out1/1
  In1/1 -> Math Function/1
  Math Function/1 -> Sum2/1
  Sum2/1 -> Sqrt/1

== system Spacecraft_ADCS (1)/Controller/Controller/PD Zenith/omega orb from orb frm to body frm ==
  In1 : Inport
  In2 : Inport  Port=2
  Math Function2 : Math  Operator=transpose  SaturateOnIntegerOverflow=on
  Product : Product  Multiplication=Matrix(*)
  q2RM1 : Subsystem
  Out1 : Outport
  wires:
  In1/1 -> q2RM1/1(In1)
  Math Function2/1 -> Product/1
  q2RM1/1(Out1) -> Math Function2/1
  In2/1 -> Product/2
  Product/1 -> Out1/1

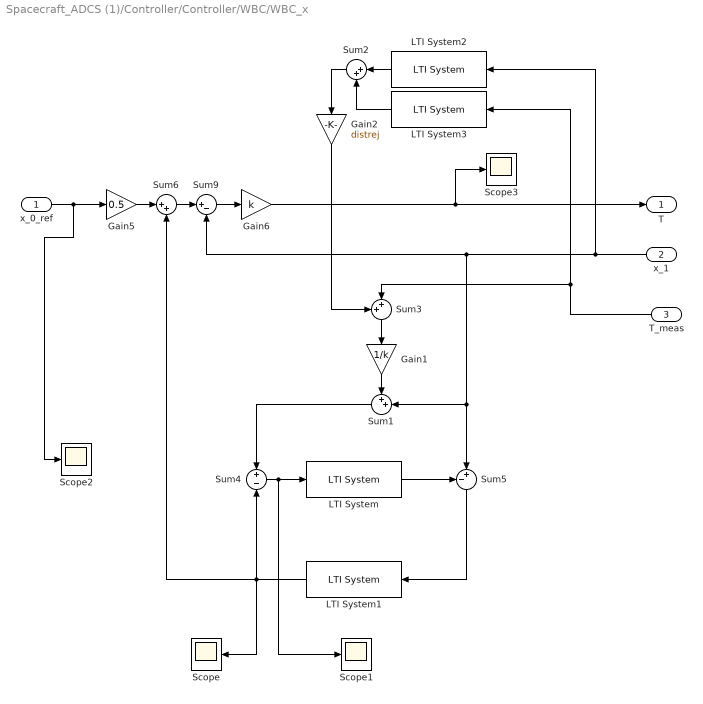
== system Spacecraft_ADCS (1)/Controller/Controller/WBC/WBC_x ==
  x_0_ref : Inport
  x_1 : Inport  Port=2
  T_meas : Inport  Port=3
  Gain1 : Gain  Gain=1/k
  Gain2 : Gain  Gain=distrej
  Gain5 : Gain  Gain=0.5
  Gain6 : Gain  Gain=k
  LTI System : cstblocks/LTI System  sys=G  IC=[]
  LTI System1 : cstblocks/LTI System  sys=G  IC=[]
  LTI System2 : cstblocks/LTI System  sys=adr(1)  IC=[]
  LTI System3 : cstblocks/LTI System  sys=adr(2)  IC=[]
  Scope{,1..3} (4 alike) : Scope
  Sum1 : Sum  Inputs=++|
  Sum2 : Sum  Inputs=|++
  Sum3 : Sum  Inputs=++|
  Sum4 : Sum  Inputs=+|-
  Sum5 : Sum  Inputs=-+|
  Sum6 : Sum  Inputs=|++
  Sum9 : Sum  Inputs=|+-
  T : Outport
  wires:
  x_0_ref/1 -> Gain5/1, Scope2/1
  T_meas/1 -> LTI System3/1, Sum3/2
  Gain2/1 -> Sum3/1
  Sum3/1 -> Gain1/1
  Sum2/1 -> Gain2/1
  LTI System3/1 -> Sum2/2
  LTI System2/1 -> Sum2/1
  Sum6/1 -> Sum9/1
  Sum9/1 -> Gain6/1
  Gain6/1 -> T/1, Scope3/1
  Gain5/1 -> Sum6/1
  LTI System1/1 -> Sum6/2, Scope/1, Sum4/2
  Sum4/1 -> LTI System/1, Scope1/1
  LTI System/1 -> Sum5/1
  Sum5/1 -> LTI System1/1
  x_1/1 -> LTI System2/1, Sum9/2, Sum5/2, Sum1/2
  Gain1/1 -> Sum1/1
  Sum1/1 -> Sum4/1

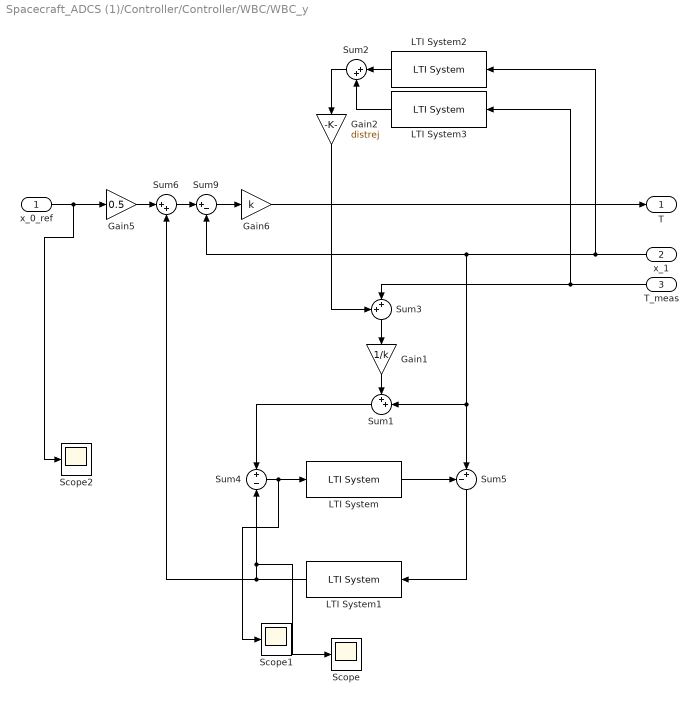
== system Spacecraft_ADCS (1)/Controller/Controller/WBC/WBC_y ==
  x_0_ref : Inport
  x_1 : Inport  Port=2
  T_meas : Inport  Port=3
  Gain1 : Gain  Gain=1/k
  Gain2 : Gain  Gain=distrej
  Gain5 : Gain  Gain=0.5
  Gain6 : Gain  Gain=k
  LTI System : cstblocks/LTI System  sys=G  IC=[]
  LTI System1 : cstblocks/LTI System  sys=G  IC=[]
  LTI System2 : cstblocks/LTI System  sys=adr(1)  IC=[]
  LTI System3 : cstblocks/LTI System  sys=adr(2)  IC=[]
  Scope : Scope
  Scope1 : Scope
  Scope2 : Scope
  Sum1 : Sum  Inputs=++|
  Sum2 : Sum  Inputs=|++
  Sum3 : Sum  Inputs=++|
  Sum4 : Sum  Inputs=+|-
  Sum5 : Sum  Inputs=-+|
  Sum6 : Sum  Inputs=|++
  Sum9 : Sum  Inputs=|+-
  T : Outport
  wires:
  Sum1/1 -> Sum4/1
  Gain1/1 -> Sum1/1
  x_1/1 -> Sum1/2, Sum5/2, Sum9/2, LTI System2/1
  Sum5/1 -> LTI System1/1
  LTI System/1 -> Sum5/1
  Sum4/1 -> Scope1/1, LTI System/1
  LTI System1/1 -> Scope/1, Sum4/2, Sum6/2
  Gain5/1 -> Sum6/1
  Gain6/1 -> T/1
  Sum9/1 -> Gain6/1
  Sum6/1 -> Sum9/1
  LTI System2/1 -> Sum2/1
  LTI System3/1 -> Sum2/2
  Sum2/1 -> Gain2/1
  Sum3/1 -> Gain1/1
  Gain2/1 -> Sum3/1
  T_meas/1 -> Sum3/2, LTI System3/1
  x_0_ref/1 -> Scope2/1, Gain5/1

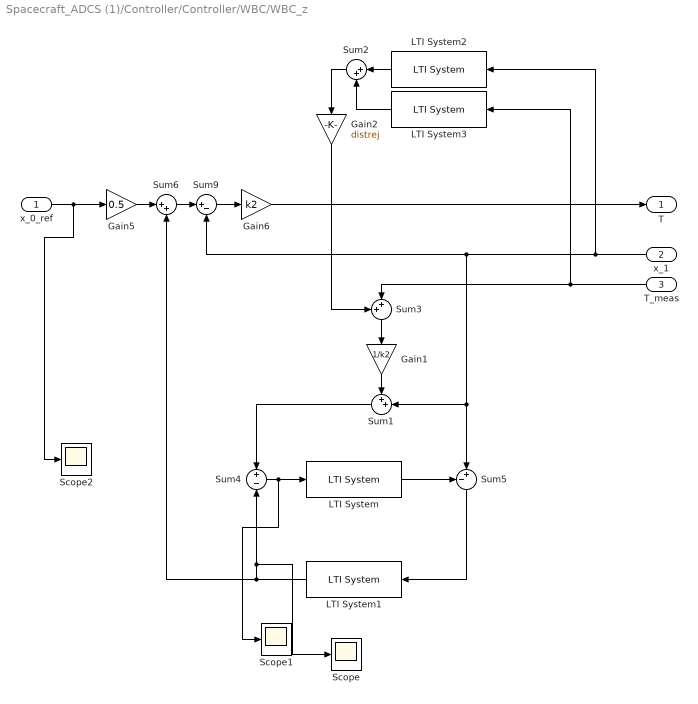
== system Spacecraft_ADCS (1)/Controller/Controller/WBC/WBC_z ==
  x_0_ref : Inport
  x_1 : Inport  Port=2
  T_meas : Inport  Port=3
  Gain1 : Gain  Gain=1/k2
  Gain2 : Gain  Gain=distrej
  Gain5 : Gain  Gain=0.5
  Gain6 : Gain  Gain=k2
  LTI System : cstblocks/LTI System  sys=G2  IC=[]
  LTI System1 : cstblocks/LTI System  sys=G2  IC=[]
  LTI System2 : cstblocks/LTI System  sys=adr2(1)  IC=[]
  LTI System3 : cstblocks/LTI System  sys=adr2(2)  IC=[]
  Scope : Scope
  Scope1 : Scope
  Scope2 : Scope
  Sum1 : Sum  Inputs=++|
  Sum2 : Sum  Inputs=|++
  Sum3 : Sum  Inputs=++|
  Sum4 : Sum  Inputs=+|-
  Sum5 : Sum  Inputs=-+|
  Sum6 : Sum  Inputs=|++
  Sum9 : Sum  Inputs=|+-
  T : Outport
  wires:
  x_0_ref/1 -> Gain5/1, Scope2/1
  T_meas/1 -> LTI System3/1, Sum3/2
  Gain2/1 -> Sum3/1
  Sum3/1 -> Gain1/1
  Sum2/1 -> Gain2/1
  LTI System3/1 -> Sum2/2
  LTI System2/1 -> Sum2/1
  Sum6/1 -> Sum9/1
  Sum9/1 -> Gain6/1
  Gain6/1 -> T/1
  Gain5/1 -> Sum6/1
  LTI System1/1 -> Sum6/2, Sum4/2, Scope/1
  Sum4/1 -> LTI System/1, Scope1/1
  LTI System/1 -> Sum5/1
  Sum5/1 -> LTI System1/1
  x_1/1 -> LTI System2/1, Sum9/2, Sum5/2, Sum1/2
  Gain1/1 -> Sum1/1
  Sum1/1 -> Sum4/1

== system Spacecraft_ADCS (1)/Controller/Controller/WBC detumble/Vector Mag1 ==
  v : Inport
  Math Function2 : Math  Operator=square  SaturateOnIntegerOverflow=on
  Sqrt2 : Sqrt  SaturateOnIntegerOverflow=on
  Sum2 : Sum  Inputs=+
  m : Outport
  wires:
  Sqrt2/1 -> m/1
  v/1 -> Math Function2/1
  Math Function2/1 -> Sum2/1
  Sum2/1 -> Sqrt2/1

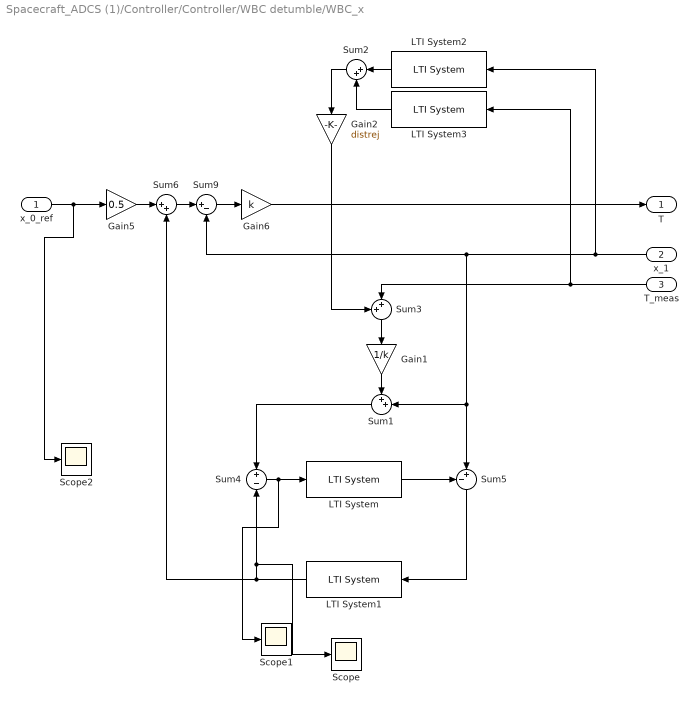
== system Spacecraft_ADCS (1)/Controller/Controller/WBC detumble/WBC_x ==
  x_0_ref : Inport
  x_1 : Inport  Port=2
  T_meas : Inport  Port=3
  Gain1 : Gain  Gain=1/k
  Gain2 : Gain  Gain=distrej
  Gain5 : Gain  Gain=0.5
  Gain6 : Gain  Gain=k
  LTI System : cstblocks/LTI System  sys=G  IC=[]
  LTI System1 : cstblocks/LTI System  sys=G  IC=[]
  LTI System2 : cstblocks/LTI System  sys=adr(1)  IC=[]
  LTI System3 : cstblocks/LTI System  sys=adr(2)  IC=[]
  Scope : Scope
  Scope1 : Scope
  Scope2 : Scope
  Sum1 : Sum  Inputs=++|
  Sum2 : Sum  Inputs=|++
  Sum3 : Sum  Inputs=++|
  Sum4 : Sum  Inputs=+|-
  Sum5 : Sum  Inputs=-+|
  Sum6 : Sum  Inputs=|++
  Sum9 : Sum  Inputs=|+-
  T : Outport
  wires:
  Sum1/1 -> Sum4/1
  Gain1/1 -> Sum1/1
  x_1/1 -> Sum1/2, Sum5/2, Sum9/2, LTI System2/1
  Sum5/1 -> LTI System1/1
  LTI System/1 -> Sum5/1
  Sum4/1 -> Scope1/1, LTI System/1
  LTI System1/1 -> Scope/1, Sum4/2, Sum6/2
  Gain5/1 -> Sum6/1
  Gain6/1 -> T/1
  Sum9/1 -> Gain6/1
  Sum6/1 -> Sum9/1
  LTI System2/1 -> Sum2/1
  LTI System3/1 -> Sum2/2
  Sum2/1 -> Gain2/1
  Sum3/1 -> Gain1/1
  Gain2/1 -> Sum3/1
  T_meas/1 -> Sum3/2, LTI System3/1
  x_0_ref/1 -> Scope2/1, Gain5/1

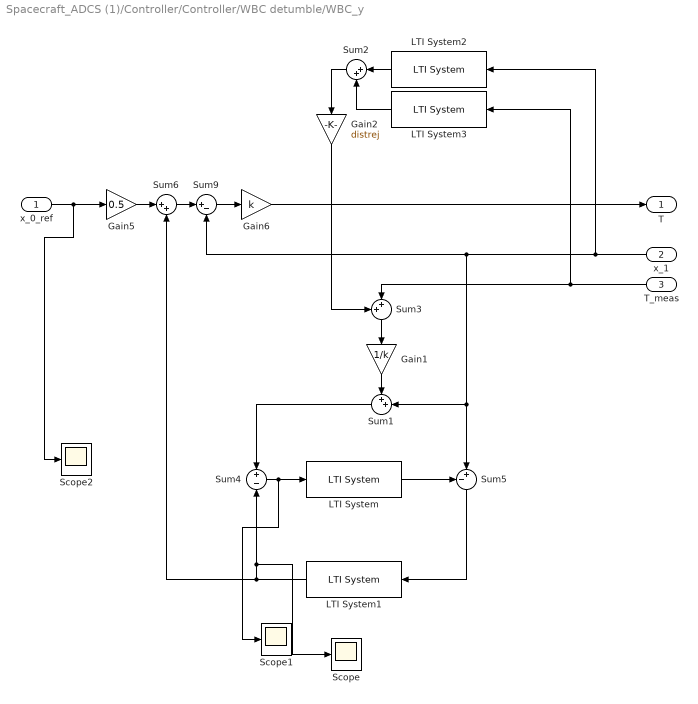
== system Spacecraft_ADCS (1)/Controller/Controller/WBC detumble/WBC_y ==
  x_0_ref : Inport
  x_1 : Inport  Port=2
  T_meas : Inport  Port=3
  Gain1 : Gain  Gain=1/k
  Gain2 : Gain  Gain=distrej
  Gain5 : Gain  Gain=0.5
  Gain6 : Gain  Gain=k
  LTI System : cstblocks/LTI System  sys=G  IC=[]
  LTI System1 : cstblocks/LTI System  sys=G  IC=[]
  LTI System2 : cstblocks/LTI System  sys=adr(1)  IC=[]
  LTI System3 : cstblocks/LTI System  sys=adr(2)  IC=[]
  Scope : Scope
  Scope1 : Scope
  Scope2 : Scope
  Sum1 : Sum  Inputs=++|
  Sum2 : Sum  Inputs=|++
  Sum3 : Sum  Inputs=++|
  Sum4 : Sum  Inputs=+|-
  Sum5 : Sum  Inputs=-+|
  Sum6 : Sum  Inputs=|++
  Sum9 : Sum  Inputs=|+-
  T : Outport
  wires:
  x_0_ref/1 -> Gain5/1, Scope2/1
  T_meas/1 -> LTI System3/1, Sum3/2
  Gain2/1 -> Sum3/1
  Sum3/1 -> Gain1/1
  Sum2/1 -> Gain2/1
  LTI System3/1 -> Sum2/2
  LTI System2/1 -> Sum2/1
  Sum6/1 -> Sum9/1
  Sum9/1 -> Gain6/1
  Gain6/1 -> T/1
  Gain5/1 -> Sum6/1
  LTI System1/1 -> Sum6/2, Sum4/2, Scope/1
  Sum4/1 -> LTI System/1, Scope1/1
  LTI System/1 -> Sum5/1
  Sum5/1 -> LTI System1/1
  x_1/1 -> LTI System2/1, Sum9/2, Sum5/2, Sum1/2
  Gain1/1 -> Sum1/1
  Sum1/1 -> Sum4/1

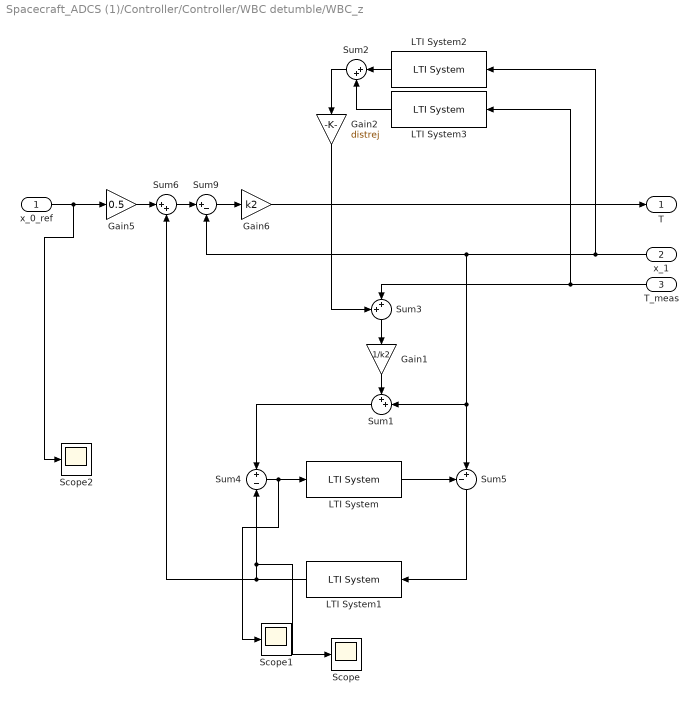
== system Spacecraft_ADCS (1)/Controller/Controller/WBC detumble/WBC_z ==
  x_0_ref : Inport
  x_1 : Inport  Port=2
  T_meas : Inport  Port=3
  Gain1 : Gain  Gain=1/k2
  Gain2 : Gain  Gain=distrej
  Gain5 : Gain  Gain=0.5
  Gain6 : Gain  Gain=k2
  LTI System : cstblocks/LTI System  sys=G2  IC=[]
  LTI System1 : cstblocks/LTI System  sys=G2  IC=[]
  LTI System2 : cstblocks/LTI System  sys=adr2(1)  IC=[]
  LTI System3 : cstblocks/LTI System  sys=adr2(2)  IC=[]
  Scope : Scope
  Scope1 : Scope
  Scope2 : Scope
  Sum1 : Sum  Inputs=++|
  Sum2 : Sum  Inputs=|++
  Sum3 : Sum  Inputs=++|
  Sum4 : Sum  Inputs=+|-
  Sum5 : Sum  Inputs=-+|
  Sum6 : Sum  Inputs=|++
  Sum9 : Sum  Inputs=|+-
  T : Outport
  wires:
  Sum1/1 -> Sum4/1
  Gain1/1 -> Sum1/1
  x_1/1 -> Sum1/2, Sum5/2, Sum9/2, LTI System2/1
  Sum5/1 -> LTI System1/1
  LTI System/1 -> Sum5/1
  Sum4/1 -> Scope1/1, LTI System/1
  LTI System1/1 -> Scope/1, Sum4/2, Sum6/2
  Gain5/1 -> Sum6/1
  Gain6/1 -> T/1
  Sum9/1 -> Gain6/1
  Sum6/1 -> Sum9/1
  LTI System2/1 -> Sum2/1
  LTI System3/1 -> Sum2/2
  Sum2/1 -> Gain2/1
  Sum3/1 -> Gain1/1
  Gain2/1 -> Sum3/1
  T_meas/1 -> Sum3/2, LTI System3/1
  x_0_ref/1 -> Scope2/1, Gain5/1

== system Spacecraft_ADCS (1)/Controller/Controller/no control/Bus ==
  In1 : Inport
  In2 : Inport  Port=2
  Bus Creator : BusCreator  Inputs=10
  Bus Selector1 : BusSelector  OutputSignals=omega_b_inert,qb_i,LongLatAlt,qb_o,qo_i,omega_orbit,T_ctrlr_meas,B_real,q_ref
  Out1 : Outport
  wires:
  Bus Selector1/9 -> Bus Creator/9  "<q_ref>"
  In2/1 -> Bus Creator/10  "T_ctrlr"
  Bus Selector1/8 -> Bus Creator/8  "<B_real>"
  Bus Selector1/7 -> Bus Creator/7  "<T_ctrlr_meas>"
  Bus Selector1/6 -> Bus Creator/6  "<omega_orbit>"
  Bus Selector1/5 -> Bus Creator/5  "<qo_i>"
  Bus Selector1/4 -> Bus Creator/4  "<qb_o>"
  Bus Selector1/3 -> Bus Creator/3  "<LongLatAlt>"
  Bus Selector1/2 -> Bus Creator/2  "<qb_i>"
  Bus Selector1/1 -> Bus Creator/1  "<omega_b_inert>"
  Bus Creator/1 -> Out1/1
  In1/1 -> Bus Selector1/1

== system Spacecraft_ADCS (1)/Actuator/Variant Subsystem/2 coil dipole/B vect from inert frm to body frm/q2RM ==
  In1 : Inport
  Add : Sum
  Constant : Constant  Value=eye(3)
  Fcn : Fcn  Commented=on  Expr=SkewSym([u(1),u(2),u(3)])
  Gain : Gain  Gain=2
  Interpreted MATLAB Function : MATLABFcn  MATLABFcn=SkewSym([u(1),u(2),u(3)],1)  OutputDimensions=9
  Math Function : Math  Operator=square  SaturateOnIntegerOverflow=on
  Product : Product
  Reshape : Reshape  OutputDimensionality=Customize  OutputDimensions=[3,3]
  Selector : Selector  InputPortWidth=4  IndexOptions=Index vector (dialog)  Indices=[1]  OutputSizes=1
  Selector1 : Selector  InputPortWidth=4  IndexOptions=Index vector (dialog)  Indices=[2 3 4]  OutputSizes=1
  Sum : Sum
  Out1 : Outport
  wires:
  Interpreted MATLAB Function/1 -> Reshape/1
  Add/1 -> Out1/1
  Constant/1 -> Add/1
  Gain/1 -> Add/2
  Sum/1 -> Gain/1
  Math Function/1 -> Sum/2
  Product/1 -> Sum/1
  Selector1/1 -> Interpreted MATLAB Function/1
  Selector/1 -> Product/1
  Reshape/1 -> Product/2, Math Function/1
  In1/1 -> Selector1/1, Selector/1

== system Spacecraft_ADCS (1)/Actuator/Variant Subsystem/3 coil dipole/B vect from inert frm to body frm/q2RM ==
  In1 : Inport
  Add : Sum
  Constant : Constant  Value=eye(3)
  Fcn : Fcn  Commented=on  Expr=SkewSym([u(1),u(2),u(3)])
  Gain : Gain  Gain=2
  Interpreted MATLAB Function : MATLABFcn  MATLABFcn=SkewSym([u(1),u(2),u(3)],1)  OutputDimensions=9
  Math Function : Math  Operator=square  SaturateOnIntegerOverflow=on
  Product : Product
  Reshape : Reshape  OutputDimensionality=Customize  OutputDimensions=[3,3]
  Selector : Selector  InputPortWidth=4  IndexOptions=Index vector (dialog)  Indices=[1]  OutputSizes=1
  Selector1 : Selector  InputPortWidth=4  IndexOptions=Index vector (dialog)  Indices=[2 3 4]  OutputSizes=1
  Sum : Sum
  Out1 : Outport
  wires:
  Interpreted MATLAB Function/1 -> Reshape/1
  Add/1 -> Out1/1
  Constant/1 -> Add/1
  Gain/1 -> Add/2
  Sum/1 -> Gain/1
  Math Function/1 -> Sum/2
  Product/1 -> Sum/1
  Selector1/1 -> Interpreted MATLAB Function/1
  Selector/1 -> Product/1
  Reshape/1 -> Product/2, Math Function/1
  In1/1 -> Selector1/1, Selector/1

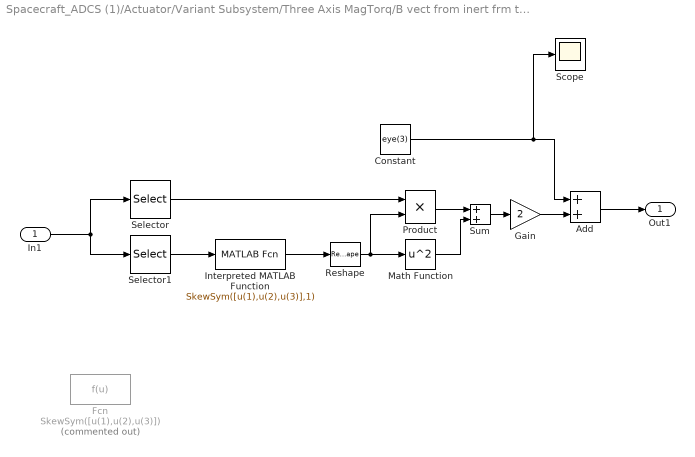
== system Spacecraft_ADCS (1)/Actuator/Variant Subsystem/Three Axis MagTorq/B vect from inert frm to body frm/q2RM2 ==
  In1 : Inport
  Add : Sum
  Constant : Constant  Value=eye(3)
  Fcn : Fcn  Commented=on  Expr=SkewSym([u(1),u(2),u(3)])
  Gain : Gain  Gain=2
  Interpreted MATLAB Function : MATLABFcn  MATLABFcn=SkewSym([u(1),u(2),u(3)],1)  OutputDimensions=9
  Math Function : Math  Operator=square  SaturateOnIntegerOverflow=on
  Product : Product
  Reshape : Reshape  OutputDimensionality=Customize  OutputDimensions=[3,3]
  Scope : Scope
  Selector : Selector  InputPortWidth=4  IndexOptions=Index vector (dialog)  Indices=[1]  OutputSizes=1
  Selector1 : Selector  InputPortWidth=4  IndexOptions=Index vector (dialog)  Indices=[2 3 4]  OutputSizes=1
  Sum : Sum
  Out1 : Outport
  wires:
  In1/1 -> Selector1/1, Selector/1
  Reshape/1 -> Math Function/1, Product/2
  Selector/1 -> Product/1
  Selector1/1 -> Interpreted MATLAB Function/1
  Product/1 -> Sum/1
  Math Function/1 -> Sum/2
  Sum/1 -> Gain/1
  Gain/1 -> Add/2
  Constant/1 -> Add/1, Scope/1
  Add/1 -> Out1/1
  Interpreted MATLAB Function/1 -> Reshape/1

== system Spacecraft_ADCS (1)/Actuator/Variant Subsystem/Three Axis MagTorq/B vect from inert frm to body frm1/q2RM2 ==
  In1 : Inport
  Add : Sum
  Constant : Constant  Value=eye(3)
  Fcn : Fcn  Commented=on  Expr=SkewSym([u(1),u(2),u(3)])
  Gain : Gain
  Interpreted MATLAB Function : MATLABFcn  MATLABFcn=SkewSym([u(1),u(2),u(3)],1)  OutputDimensions=9
  Math Function : Math  Operator=square  SaturateOnIntegerOverflow=on
  Product : Product
  Reshape : Reshape  OutputDimensionality=Customize  OutputDimensions=[3,3]
  Selector : Selector  InputPortWidth=4  IndexOptions=Index vector (dialog)  Indices=[1]  OutputSizes=1
  Selector1 : Selector  InputPortWidth=4  IndexOptions=Index vector (dialog)  Indices=[2 3 4]  OutputSizes=1
  Sum : Sum
  Out1 : Outport
  wires:
  Interpreted MATLAB Function/1 -> Reshape/1
  Add/1 -> Out1/1
  Constant/1 -> Add/1
  Gain/1 -> Add/2
  Sum/1 -> Gain/1
  Math Function/1 -> Sum/2
  Product/1 -> Sum/1
  Selector1/1 -> Interpreted MATLAB Function/1
  Selector/1 -> Product/1
  Reshape/1 -> Product/2, Math Function/1
  In1/1 -> Selector1/1, Selector/1

== system Spacecraft_ADCS (1)/Controller/Controller/PD Zenith/B vect from inert frm to body frm/q2RM2 ==
  In1 : Inport
  Add : Sum
  Constant : Constant  Value=eye(3)
  Fcn : Fcn  Commented=on  Expr=SkewSym([u(1),u(2),u(3)])
  Gain : Gain  Gain=2
  Interpreted MATLAB Function : MATLABFcn  MATLABFcn=SkewSym([u(1),u(2),u(3)],1)  OutputDimensions=9
  Math Function : Math  Operator=square  SaturateOnIntegerOverflow=on
  Product : Product
  Reshape : Reshape  OutputDimensionality=Customize  OutputDimensions=[3,3]
  Selector : Selector  InputPortWidth=4  IndexOptions=Index vector (dialog)  Indices=[1]  OutputSizes=1
  Selector1 : Selector  InputPortWidth=4  IndexOptions=Index vector (dialog)  Indices=[2 3 4]  OutputSizes=1
  Sum : Sum
  Out1 : Outport
  wires:
  In1/1 -> Selector/1, Selector1/1
  Reshape/1 -> Math Function/1, Product/2
  Selector/1 -> Product/1
  Selector1/1 -> Interpreted MATLAB Function/1
  Product/1 -> Sum/1
  Math Function/1 -> Sum/2
  Sum/1 -> Gain/1
  Gain/1 -> Add/2
  Constant/1 -> Add/1
  Add/1 -> Out1/1
  Interpreted MATLAB Function/1 -> Reshape/1

== system Spacecraft_ADCS (1)/Controller/Controller/PD Zenith/omega orb from orb frm to body frm/q2RM1 ==
  In1 : Inport
  Add : Sum
  Constant : Constant  Value=eye(3)
  Fcn : Fcn  Commented=on  Expr=SkewSym([u(1),u(2),u(3)])
  Gain : Gain  Gain=2
  Interpreted MATLAB Function : MATLABFcn  MATLABFcn=SkewSym([u(1),u(2),u(3)],1)  OutputDimensions=9
  Math Function : Math  Operator=square  SaturateOnIntegerOverflow=on
  Product : Product
  Reshape : Reshape  OutputDimensionality=Customize  OutputDimensions=[3,3]
  Selector : Selector  InputPortWidth=4  IndexOptions=Index vector (dialog)  Indices=[1]  OutputSizes=1
  Selector1 : Selector  InputPortWidth=4  IndexOptions=Index vector (dialog)  Indices=[2 3 4]  OutputSizes=1
  Sum : Sum
  Out1 : Outport
  wires:
  Interpreted MATLAB Function/1 -> Reshape/1
  Add/1 -> Out1/1
  Constant/1 -> Add/1
  Gain/1 -> Add/2
  Sum/1 -> Gain/1
  Math Function/1 -> Sum/2
  Product/1 -> Sum/1
  Selector1/1 -> Interpreted MATLAB Function/1
  Selector/1 -> Product/1
  Reshape/1 -> Product/2, Math Function/1
  In1/1 -> Selector1/1, Selector/1
